simulink model "cw7_model_Gajda"  (R2017b)
settings: Solver=VariableStepAuto  StartTime=0.0  StopTime=500  MaxStep=0.01  MinStep=0.001  RelTol=1e-6
values from neighbouring files (symbols this model uses):
  a0 = 1/(R1*C1)    (= 0.2)    [cw7_dane_Gajda.m]
  a1 = 1/C1    (= 0.1)    [cw7_dane_Gajda.m]
  b0 = 1/(R1*C2)    (= 0.4)    [cw7_dane_Gajda.m]
  b1 = 1/(R2*C2)    (= 0.1)    [cw7_dane_Gajda.m]
  p0 = x20    (= 2)    [cw7_dane_Gajda.m]
  x10 = 2.5    [cw7_dane_Gajda.m]
  x20 = 2    [cw7_dane_Gajda.m]
settings Model: Creator=MG  LastModifiedBy=MG
settings DataIOCC: SaveFormat=Array

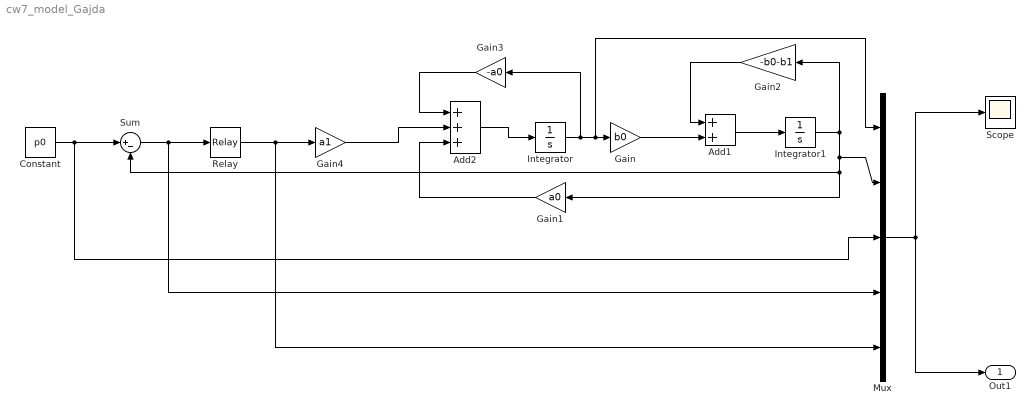
== system cw7_model_Gajda ==
  Add1 : Sum
  Add2 : Sum  Inputs=+++
  Constant : Constant  Value=p0
  Gain : Gain  Gain=b0
  Gain1 : Gain  Gain=a0
  Gain2 : Gain  Gain=-b0-b1
  Gain3 : Gain  Gain=-a0
  Gain4 : Gain  Gain=a1
  Integrator : Integrator  InitialCondition=x10
  Integrator1 : Integrator  InitialCondition=x20
  Mux : Mux  Inputs=5
  Relay : Relay  OffSwitchValue=-eps  OnOutputValue=U
  Scope : Scope
  Sum : Sum  Inputs=|+-
  Out1 : Outport  VectorParamsAs1DForOutWhenUnconnected=on
  wires:
  Integrator/1 -> Gain3/1, Mux/1, Gain/1
  Constant/1 -> Mux/3, Sum/1
  Gain3/1 -> Add2/1
  Integrator1/1 -> Sum/2, Gain1/1, Mux/2, Gain2/1
  Gain4/1 -> Add2/2
  Gain2/1 -> Add1/1
  Add2/1 -> Integrator/1
  Sum/1 -> Mux/4, Relay/1
  Gain1/1 -> Add2/3
  Mux/1 -> Scope/1, Out1/1
  Add1/1 -> Integrator1/1
  Gain/1 -> Add1/2
  Relay/1 -> Mux/5, Gain4/1
